simulink model "FLC_Cotroller"  (R2014a)
settings: Solver=ode45  StartTime=0.0  StopTime=10.0  RelTol=1e-3
libraries: fuzblock x1
settings Model: Creator=mamta  LastModifiedBy=mamta
settings SolverCC: ZeroCrossAlgorithm=Adaptive

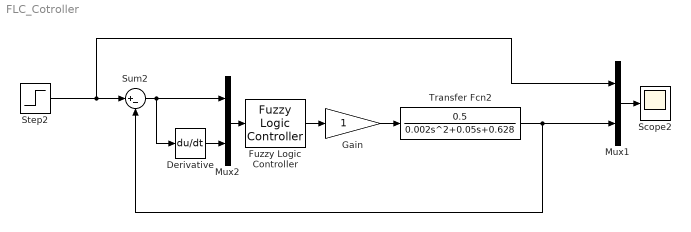
== system FLC_Cotroller ==
  Derivative : Derivative
  Fuzzy Logic Controller : fuzblock/Fuzzy Logic  Controller  fis='singam'
  Gain : Gain
  Mux1 : Mux  Inputs=2
  Mux2 : Mux  Inputs=2
  Scope2 : Scope
      settings: YMin=0.9935  YMax=1
  Step2 : Step  SampleTime=0
  Sum2 : Sum  Inputs=|+-
  Transfer Fcn2 : TransferFcn  Numerator=[0.5]  Denominator=[0.002 0.05 0.628]
  wires:
  Step2/1 -> Mux1/1, Sum2/1
  Sum2/1 -> Mux2/1, Derivative/1
  Mux1/1 -> Scope2/1
  Derivative/1 -> Mux2/2
  Mux2/1 -> Fuzzy Logic Controller/1
  Fuzzy Logic Controller/1 -> Gain/1
  Transfer Fcn2/1 -> Mux1/2, Sum2/2
  Gain/1 -> Transfer Fcn2/1
